simulink model "bike"  (R2018b)
settings: Solver=VariableStepAuto  StartTime=0.0  StopTime=10.0  RelTol=1e-3
values from neighbouring files (symbols this model uses):
  A = [0    m*g*h_real/J ... (first row only)    [UncertaintyPlot_new.m]
  b = 1.095    [report_gutman.m]
  B = [1; 0]    [UncertaintyPlot_new.m]
  bike_params = [g h b a lambda m]    [report_gutman.m]
  C = [v*D_inertia/(b_real*J) m*v^2*h_real/(b_real*J)]    [UncertaintyPlot_new.m]
  D = 0    [UncertaintyPlot_new.m]
  IMU_height = 0.45    [report_gutman.m]
  initial_roll = deg2rad(2)    [report_gutman.m]
  initial_rollrate = deg2rad(2)    [report_gutman.m]
  lambda = deg2rad(70)    [report_gutman.m]
  Ts = 0.04    [UncertaintyPlot_new.m]    (also in report_gutman.m = 0.01)
  v = 5    [UncertaintyPlot_new.m]    (also in bike_linear_analysis2.m = v_vec(i); bike_pd_linear_analysis.m = 4; bike_pd_steering_linear_analysis.m = 4; bike_pd_steering_linear_analysis2.m = 4)
settings Model: Creator=maximef  LastModifiedBy=maximef

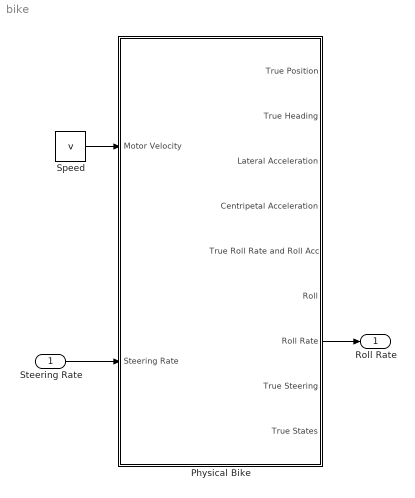
== system bike ==
  Steering Rate : Inport
  Physical Bike : Subsystem
  Speed : Constant  Value=v
  Roll Rate : Outport
  wires:
  Speed/1 -> Physical Bike/1(Motor Velocity)
  Physical Bike/7(Roll Rate) -> Roll Rate/1
  Steering Rate/1 -> Physical Bike/2(Steering Rate)

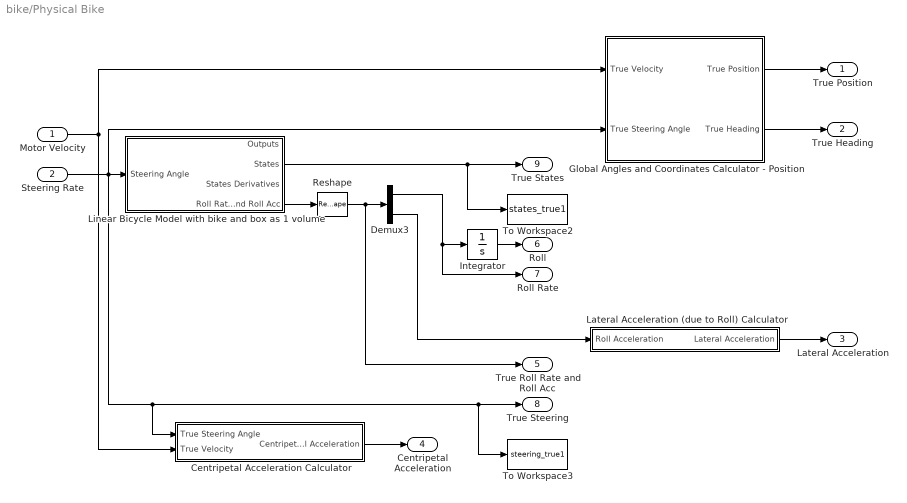
== system bike/Physical Bike ==
  Motor Velocity : Inport
  Steering Rate : Inport  Port=2
  Centripetal Acceleration Calculator : Subsystem
  Demux3 : Demux  Outputs=2
  Global Angles and Coordinates Calculator - Position : Subsystem  SystemSampleTime=Ts
  Integrator : Integrator  InitialCondition=initial_roll
  Lateral Acceleration (due to Roll) Calculator : Subsystem
  Linear Bicycle Model with bike and box as 1 volume : Subsystem
  Reshape : Reshape
  To Workspace2 : ToWorkspace  VariableName=states_true1  SaveFormat=Timeseries  SampleTime=-1
  To Workspace3 : ToWorkspace  VariableName=steering_true1  SaveFormat=Timeseries  SampleTime=-1
  True Position : Outport
  True Heading : Outport  Port=2
  Lateral Acceleration : Outport  Port=3
  Centripetal Acceleration : Outport  Port=4
  True Roll Rate and Roll Acc : Outport  Port=5
  Roll : Outport  Port=6
  Roll Rate : Outport  Port=7
  True Steering : Outport  Port=8
  True States : Outport  Port=9
  wires:
  Steering Rate/1 -> Global Angles and Coordinates Calculator - Position/2(True Steering Angle), To Workspace3/1, True Steering/1, Centripetal Acceleration Calculator/1(True Steering Angle), Linear Bicycle Model with bike and box as 1 volume/1(Steering Angle)
  Centripetal Acceleration Calculator/1(Centripetal Acceleration) -> Centripetal Acceleration/1
  Demux3/2 -> Lateral Acceleration (due to Roll) Calculator/1(Roll Acceleration)
  Lateral Acceleration (due to Roll) Calculator/1(Lateral Acceleration) -> Lateral Acceleration/1
  Linear Bicycle Model with bike and box as 1 volume/2(States) -> To Workspace2/1, True States/1
  Demux3/1 -> Integrator/1, Roll Rate/1
  Reshape/1 -> True Roll Rate and Roll Acc/1, Demux3/1
  Linear Bicycle Model with bike and box as 1 volume/4(Roll Rate and Roll Acc) -> Reshape/1
  Motor Velocity/1 -> Centripetal Acceleration Calculator/2(True Velocity), Global Angles and Coordinates Calculator - Position/1(True Velocity)
  Global Angles and Coordinates Calculator - Position/1(True Position) -> True Position/1
  Global Angles and Coordinates Calculator - Position/2(True Heading) -> True Heading/1
  Integrator/1 -> Roll/1

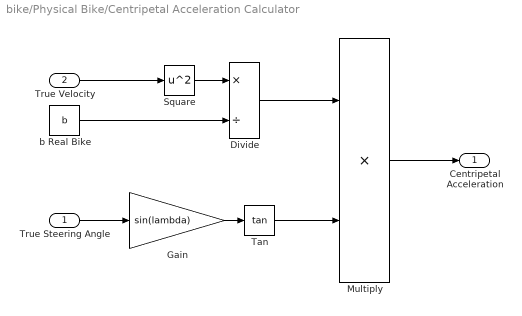
== system bike/Physical Bike/Centripetal Acceleration Calculator ==
  True Steering Angle : Inport
  True Velocity : Inport  Port=2
  Divide : Product  Inputs=*/
  Gain : Gain  Gain=sin(lambda)
  Multiply : Product
  Square : Math  Operator=square  SaturateOnIntegerOverflow=on
  Tan : Trigonometry  Operator=tan
  b Real Bike : Constant  Value=b
  Centripetal Acceleration : Outport
  wires:
  True Velocity/1 -> Square/1
  Square/1 -> Divide/1
  b Real Bike/1 -> Divide/2
  True Steering Angle/1 -> Gain/1
  Divide/1 -> Multiply/1
  Tan/1 -> Multiply/2
  Multiply/1 -> Centripetal Acceleration/1
  Gain/1 -> Tan/1

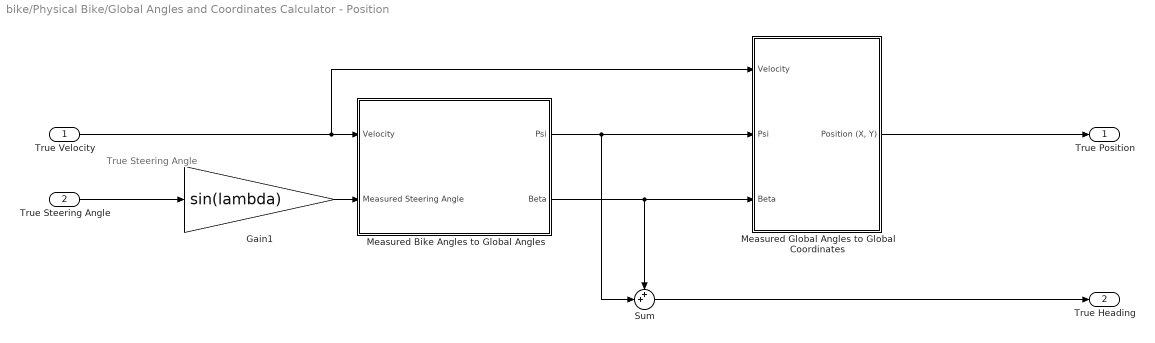
== system bike/Physical Bike/Global Angles and Coordinates Calculator - Position ==
  note: True Steering
      | Angle
  True Velocity : Inport
  True Steering Angle : Inport  Port=2
  Gain1 : Gain  Gain=sin(lambda)
  Measured Bike Angles to Global Angles : Subsystem
  Measured Global Angles to Global Coordinates : Subsystem
  Sum : Sum  Inputs=++|
  True Position : Outport
  True Heading : Outport  Port=2
  wires:
  Measured Bike Angles to Global Angles/1(Psi) -> Sum/2, Measured Global Angles to Global Coordinates/2(Psi)
  Gain1/1 -> Measured Bike Angles to Global Angles/2(Measured Steering Angle)
  Sum/1 -> True Heading/1
  Measured Bike Angles to Global Angles/2(Beta) -> Sum/1, Measured Global Angles to Global Coordinates/3(Beta)
  Measured Global Angles to Global Coordinates/1("Position (X, Y)") -> True Position/1
  True Velocity/1 -> Measured Global Angles to Global Coordinates/1(Velocity), Measured Bike Angles to Global Angles/1(Velocity)
  True Steering Angle/1 -> Gain1/1

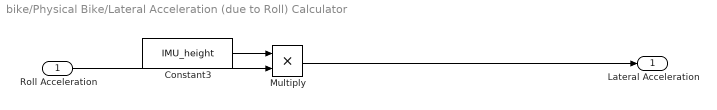
== system bike/Physical Bike/Lateral Acceleration (due to Roll) Calculator ==
  Roll Acceleration : Inport
  Constant3 : Constant  Value=IMU_height
  Multiply : Product
  Lateral Acceleration : Outport
  wires:
  Multiply/1 -> Lateral Acceleration/1
  Constant3/1 -> Multiply/1
  Roll Acceleration/1 -> Multiply/2

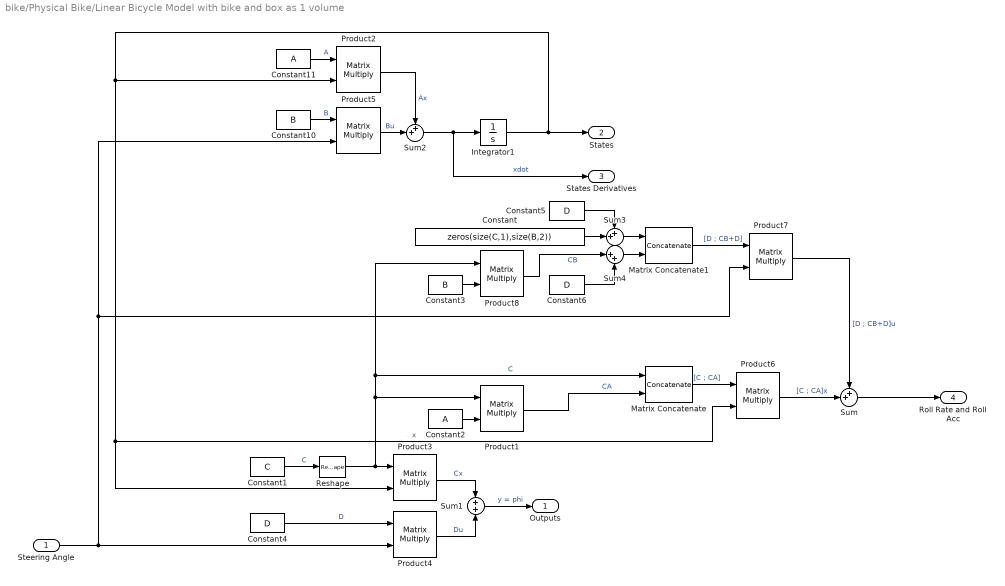
== system bike/Physical Bike/Linear Bicycle Model with bike and box as 1 volume ==
  Steering Angle : Inport
  Constant : Constant  Value=zeros(size(C,1),size(B,2))
  Constant1 : Constant  Value=C
  Constant10 : Constant  Value=B
  Constant11 : Constant  Value=A
  Constant2 : Constant  Value=A
  Constant3 : Constant  Value=B
  Constant4 : Constant  Value=D
  Constant5 : Constant  Value=D
  Constant6 : Constant  Value=D
  Integrator1 : Integrator  InitialCondition=[C ; C*A]\[initial_rollrate ; 0]
  Matrix Concatenate : Concatenate  Mode=Multidimensional array
  Matrix Concatenate1 : Concatenate  Mode=Multidimensional array
  Product{1..8} (8 alike) : Product  SCDEnableBlockLinearizationSpecification=on  Multiplication=Matrix(*)
  Reshape : Reshape  OutputDimensionality=Customize  OutputDimensions=[size(C,1),size(C,2)]
  Sum : Sum  Inputs=++|
  Sum1 : Sum
  Sum2 : Sum  Inputs=++|
  Sum3 : Sum  Inputs=++|
  Sum4 : Sum  Inputs=|++
  Outputs : Outport
  States : Outport  Port=2
  States Derivatives : Outport  Port=3
  Roll Rate and Roll Acc : Outport  Port=4
  wires:
  Reshape/1 -> Product3/1, Product8/1, Matrix Concatenate/1, Product1/1  "C"
  Sum/1 -> Roll Rate and Roll Acc/1
  Constant1/1 -> Reshape/1  "C"
  Matrix Concatenate/1 -> Product6/1  "[C ; CA]"
  Product5/1 -> Sum2/2  "Bu"
  Matrix Concatenate1/1 -> Product7/1  "[D ; CB+D]"
  Constant11/1 -> Product2/1  "A"
  Constant3/1 -> Product8/2
  Product6/1 -> Sum/2  "[C ; CA]x"
  Sum2/1 -> Integrator1/1, States Derivatives/1  "xdot"
  Product2/1 -> Sum2/1  "Ax"
  Product1/1 -> Matrix Concatenate/2  "CA"
  Product8/1 -> Sum4/1  "CB"
  Integrator1/1 -> Product2/2, Product6/2, Product3/2, States/1  "x"
  Sum1/1 -> Outputs/1  "y = phi"
  Constant2/1 -> Product1/2
  Product7/1 -> Sum/1  "[D ; CB+D]u"
  Constant10/1 -> Product5/1  "B"
  Steering Angle/1 -> Product4/2, Product5/2, Product7/2
  Product4/1 -> Sum1/2  "Du"
  Product3/1 -> Sum1/1  "Cx"
  Constant4/1 -> Product4/1  "D"
  Sum3/1 -> Matrix Concatenate1/1
  Constant/1 -> Sum3/2
  Constant5/1 -> Sum3/1
  Sum4/1 -> Matrix Concatenate1/2
  Constant6/1 -> Sum4/2

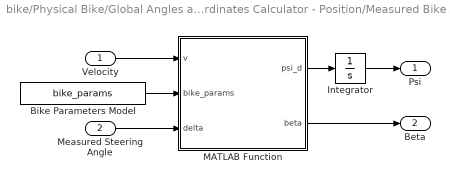
== system bike/Physical Bike/Global Angles and Coordinates Calculator - Position/Measured Bike Angles to Global Angles ==
  Velocity : Inport
  Measured Steering Angle : Inport  Port=2
  " Bike Parameters Model " : Constant  Value=bike_params
  Integrator : Integrator
  MATLAB Function : MATLAB Function  TreatAsAtomicUnit=on
  Psi : Outport
  Beta : Outport  Port=2
  wires:
  MATLAB Function/2(beta) -> Beta/1
  MATLAB Function/1(psi_d) -> Integrator/1
  Integrator/1 -> Psi/1
  " Bike Parameters Model "/1 -> MATLAB Function/2(bike_params)
  Measured Steering Angle/1 -> MATLAB Function/3(delta)
  Velocity/1 -> MATLAB Function/1(v)

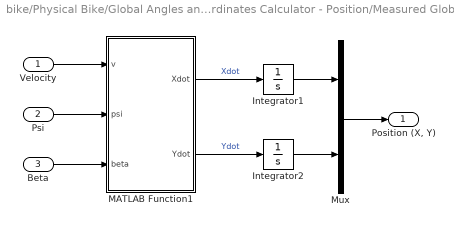
== system bike/Physical Bike/Global Angles and Coordinates Calculator - Position/Measured Global Angles to Global Coordinates ==
  Velocity : Inport
  Psi : Inport  Port=2
  Beta : Inport  Port=3
  Integrator1 : Integrator
  Integrator2 : Integrator
  MATLAB Function1 : MATLAB Function  TreatAsAtomicUnit=on
  Mux : Mux  Inputs=2
  "Position (X, Y)" : Outport
  wires:
  MATLAB Function1/2(Ydot) -> Integrator2/1  "Ydot"
  MATLAB Function1/1(Xdot) -> Integrator1/1  "Xdot"
  Psi/1 -> MATLAB Function1/2(psi)
  Beta/1 -> MATLAB Function1/3(beta)
  Velocity/1 -> MATLAB Function1/1(v)
  Integrator2/1 -> Mux/2
  Integrator1/1 -> Mux/1
  Mux/1 -> "Position (X, Y)"/1

== matlab function bike/Physical Bike/Global Angles and Coordinates Calculator - Position/Measured Bike Angles to Global Angles/MATLAB Function ==
  data: v input; bike_params input; delta input; psi_d output; beta output
function [psi_d, beta]  = fcn(v, bike_params, delta)

b = bike_params(3);
a = bike_params(4);

beta = atan((a / (b)) * tan(delta));
psi_d = (v / a) * sin(beta);

== matlab function bike/Physical Bike/Global Angles and Coordinates Calculator - Position/Measured Global Angles to Global Coordinates/MATLAB Function1 ==
  data: v input; psi input; Xdot output; beta input; Ydot output
function [Xdot, Ydot]  = fcn(v, psi, beta)

Xdot = v * cos(psi + beta);
Ydot = v * sin(psi + beta);
